simulink model "Final_System_Model_V2"  (R2018a)
settings: Solver=VariableStepAuto  StartTime=0  StopTime=inf  RelTol=1e-3
PreLoadFcn:
  | Ts_Power=1e-6;
  | Ts_Control=100e-6;
undefined symbols (not defined in the file): DiscIntNeverNeededParam, FC, FuelCellLoadFcn, gcbh, Ion, Lithium, sigbuilder_block, sps_rtmsupport
libraries: powerlib x20, simulink x10, fl_lib x8, nesl_utility x6, powerlib_meascontrol x5, electricdrivelib x1, spsFuelCellModel x1, re_lib x1
(part 1 of 4)
Description:
  | Copyright 2008-2017 The MathWorks, Inc.
settings Model: SimulationMode=accelerator  PacingRate=0.400000  Creator=MathWorks  LastModifiedBy=Mina
settings SolverCC: ZeroCrossControl=EnableAll  ZeroCrossAlgorithm=Adaptive  AlgebraicLoopSolver=LineSearch
settings DataIOCC: LimitDataPoints=on  SaveFormat=Array  SignalLoggingSaveFormat=ModelDataLogs  SignalLogging=off  DSMLogging=off
settings OptimizationCC: ExpressionDepthLimit=2147483647  LifeSpan=inf
settings DebuggingCC: SolverPrmCheckMsg=warning  FcnCallInpInsideContextMsg=warning  StateNameClashWarn=warning  SFUnexpectedBacktrackingDiag=warning  SFNoUnconditionalDefaultTransitionDiag=warning  SFExecutionAtInitializationDiag=none
settings HardwareCC: ProdBitPerPointer=32  ProdBitPerSizeT=32  ProdBitPerPtrDiffT=32  ProdLargestAtomicFloat=None  ProdIntDivRoundTo=Undefined  ProdEndianess=Unspecified  ProdWordSize=32  ProdHWDeviceType=32-bit Generic
settings ModelReferenceCC: PropagateSignalLabelsOutOfModel=off
settings CodeAppCC: StateflowObjectComments=on
settings GRTTargetCC: TargetLangStandard=C89/C90 (ANSI)  GeneratePreprocessorConditionals=Disable all  CombineOutputUpdateFcns=off  GRTInterface=on
settings ConfigComp: CovMetricSettings=dw  CovHtmlReporting=on  CovSaveCumulativeToWorkspaceVar=on  CovSaveSingleToWorkspaceVar=on  CovExternalEMLEnable=off  CovSFcnEnable=off
settings SimscapeCC: SimscapeNormalizeSystem=off

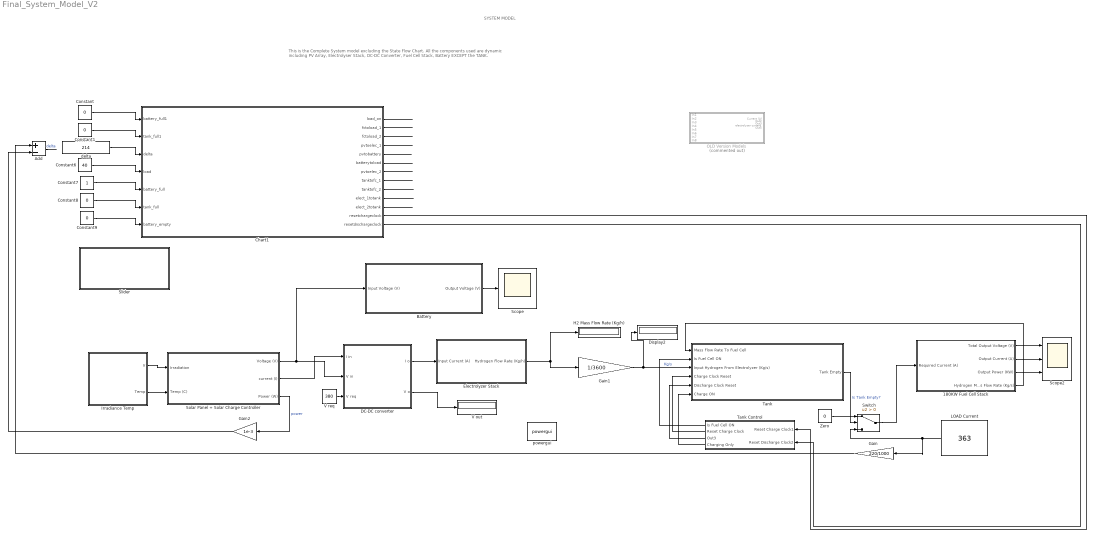
== system Final_System_Model_V2 ==
  note: SYSTEM MODEL
  note: This is the Complete System model excluding the State Flow Chart.
      |
      | All the components used are dynamic including PV Array, Electrolyser Stack, DC-DC Converter, Fuel Cell Stack, Battery EXCEPT the TANK.
  180KW Fuel Cell Stack : Subsystem
  Add : Sum  Inputs=+-
  Battery : Subsystem
  Chart1 : Stateflow chart  TreatAsAtomicUnit=on
  Constant{,1,8..9} (4 alike) : Constant  Value=0
  Constant6 : Constant  Value=40
  Constant7 : Constant
  DC-DC converter : Subsystem
  Display2 : Display
  Electrolyzer Stack : Subsystem
  Gain : Gain  Gain=220/1000
  Gain1 : Gain  Gain=1/3600
  Gain2 : Gain  Gain=1e-3
  H2 Mass Flow Rate (Kg/h) : Display
      settings: Format=short_e  Decimation=1000
  Irradiance Temp : Subsystem  Tag=STV Subsys  LoadFcn=sigbuilder_block('load');  StartFcn=sigbuilder_block('start');  StopFcn=sigbuilder_block('stop');  ClipboardFcn=sigbuilder_block('clipboard');  mask(Sigbuilder block){tuvar=[0:10]}
      mask help: Sigbuilder GUI
      mask init:
      | if ~strcmp(get_param(bdroot(gcbh),'SimulationStatus'),'stopped') tuvar = sigbuilder_block('maskInit'); end
      settings: CopyFcn=sigbuilder_block('copy');  DeleteFcn=sigbuilder_block('delete');  ModelCloseFcn=sigbuilder_block('modelClose');  PreSaveFcn=sigbuilder_block('preSave');  PauseFcn=sigbuilder_block('pause')  ContinueFcn=sigbuilder_block('continue')  NameChangeFcn=sigbuilder_block('namechange');  OpenFcn=sigbuilder_block('open',[216.75 189 451.5 323.25 ]);  CloseFcn=sigbuilder_block('close');
      mask Display: plot(0, 0, 100, 100,[2, 2, 32, 32, 2], [68, 8, 8, 68, 68],[32, 2], [38, 38], [32, 19, 2],[53, 60, 44], [32, 17, 17, 2],[16, 16, 31, 31]);txt = getActiveGroup(gcbh);text(2, 100, txt,'verticalAlignment', 'top');
  LOAD Current : Constant  Value=363
  OLD Version Models : Subsystem  Commented=on
  Scope : Scope
  Scope2 : Scope  NumInputPorts=3
  Slider : Subsystem  DialogController=hmiCreateDDGDialog  IsWebBlock=on  mask(MWDashboardBlock){webBlockId=9211a712-9074-4bf0-88da-f75de64371df, webBlockType=slider, ShowInLibBrowser=on, ShowInitialText=on, HMISrcModelName=Final_System_Model_V2}
      mask prompts: webBlockId "WebBlock Id"; webBlockType "WebBlock Type"; HMISrcModelName "Source Model"
      mask help: SimulinkHMI:dialogs:SliderDialogDesc
      mask Help: helpview([docroot '/mapfiles/simulink.map'], 'hmi_slider')
      mask Display:
      | if strcmp(get_param(bdroot(gcb),'BlockDiagramType'), 'library')
      |     image([(matlabroot) '/toolbox/simulink/hmi/icons/Slider.png']);
      | end
  Solar Panel + Solar Charge Controller : Subsystem
  Switch : Switch  Criteria=u2 > Threshold
  Tank : Subsystem
  Tank Control : Subsystem
  V out : Display
  V req : Constant  Value=380
  Zero : Constant  Value=0
  delta : Constant  Value=214
  powergui : powerlib/powergui  Priority=1  SimulationMode=Discrete  SampleTime=50e-6  frequency=60  Iterations=50  frequencyindice=0  Pbase=100e6  ErrMax=1e-4  UnitsV=kV  UnitsW=MW  buscounter=0  FunctionMessages=off  echomessages=off  EnableUseOfTLC=off  CurrentSourceSwitches=off  DisableSnubberDevices=off  DisableRonSwitches=off  DisableVfSwitches=off  DisplayEquations=off  SolverType=Tustin/Backward Euler (TBE)  Interpol=off  ExternalGateDelay=off  methode=off  Ts=100  x0status=blocks  SPID=off  SwTol=0  HookPort=off  RestoreLinks=warning  ResistiveCurrentMeasurement=off  Frange=[0:2:500]  Ylog=off  Xlog=on  ShowGrid=off  save=off  variable=ZData  structure=0  ZoomFFT=off  StartTime=0.0  cycles=1  DisplayStyle=1  fundamental=60  FreqAxis=off  MaxFrequency=1000  frequencyindicesteady=1  RmsSteady=1  display=off
  wires:
  Irradiance Temp/1(Ir) -> Solar Panel + Solar Charge Controller/1(Irradiation)
  Irradiance Temp/2(Temp) -> Solar Panel + Solar Charge Controller/2(Temp (C))
  Battery/1(Output Voltage (V)) -> Scope/1
  Electrolyzer Stack/1(Hydrogen Flow Rate (Kg/h)) -> H2 Mass Flow Rate (Kg/h)/1, Gain1/1
  180KW Fuel Cell Stack/1(Total Output Voltage (V)) -> Scope2/1
  180KW Fuel Cell Stack/2(Output Current (A)) -> Scope2/2
  180KW Fuel Cell Stack/3(Output Power (KW)) -> Scope2/3
  Gain1/1 -> Display2/1, Tank/3(Input Hydrogen From Electrolyzer (Kg/s))  "Kg/s"
  LOAD Current/1 -> Gain/1, Switch/3
  Solar Panel + Solar Charge Controller/3(Power (W)) -> Gain2/1  "power"
  180KW Fuel Cell Stack/4(Hydrogen Mass Flow Rate (Kg/s)) -> Tank/1(Mass Flow Rate To Fuel Cell)
  Tank/1(Tank Empty) -> Switch/2  "Is Tank Empty?"
  V req/1 -> DC-DC converter/3(V req)
  Solar Panel + Solar Charge Controller/1(Voltage (V)) -> DC-DC converter/2(V in), Battery/1(Input Voltage (V))
  DC-DC converter/1(I o) -> Electrolyzer Stack/1(Input Current (A))
  Solar Panel + Solar Charge Controller/2(current (I)) -> DC-DC converter/1(I in)
  DC-DC converter/2(V o) -> V out/1
  Tank Control/1(Is Fuel Cell ON) -> Tank/2(Is Fuel Cell ON)
  Tank Control/2(Reset Charge Clock) -> Tank/4(Charge Clock Reset)
  Tank Control/3(Out3) -> Tank/5(Discharge Clock Reset)
  Tank Control/4(Charging Only) -> Tank/6(Charge ON)
  Switch/1 -> 180KW Fuel Cell Stack/1(Required Current (A))
  Zero/1 -> Switch/1
  Gain/1 -> Add/1
  Gain2/1 -> Add/2
  Add/1 -> ?  "delta"
  Constant/1 -> Chart1/1(battery_full1)
  Constant1/1 -> Chart1/2(tank_full1)
  delta/1 -> Chart1/3(delta)
  Constant6/1 -> Chart1/4(load)
  Constant7/1 -> Chart1/5(battery_full)
  Constant8/1 -> Chart1/6(tank_full)
  Constant9/1 -> Chart1/7(battery_empty)
  Chart1/1(load_on) -> ?
  Chart1/2(fctoload_1) -> ?
  Chart1/3(fctoload_2) -> ?
  Chart1/4(pvtoelec_1) -> ?
  Chart1/5(pvtobattery) -> ?
  Chart1/6(batterytoload) -> ?
  Chart1/7(pvtoelec_2) -> ?
  Chart1/8(tanktofc_1) -> ?
  Chart1/9(tanktofc_2) -> ?
  Chart1/10(elect_1totank) -> ?
  Chart1/11(elect_2totank) -> ?
  Chart1/12(resetchargeclock) -> Tank Control/1(Reset Charge Clock1)
  Chart1/13(resetdischargeclock) -> Tank Control/2(Reset Discharge Clock2)

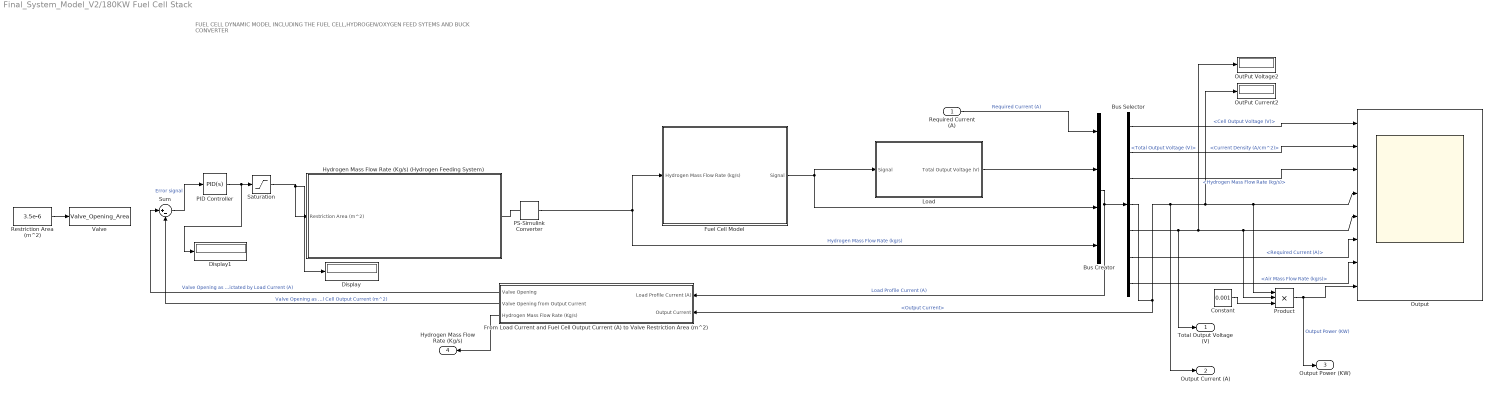
== system Final_System_Model_V2/180KW Fuel Cell Stack ==
  note: FUEL CELL DYNAMIC MODEL INCLUDING THE FUEL CELL,HYDROGEN/OXYGEN FEED SYTEMS AND BUCK CONVERTER
  Required Current (A) : Inport
  Bus Creator : BusCreator  Inputs=4
  Bus Selector : BusSelector  OutputSignals=|
      | signal3.Cell Output Voltage (V),signal3.Current Density (A/cm^2),Hydrogen Mass Flow Rate (kg/s),signal3.Output Current,Total Output Voltage (V),Required Current
      | (A),signal3.Air Mass Flow Rate (kg/s)
  Constant : Constant  Value=0.001
  Display : Display
  Display1 : Display
  From Load Current and Fuel Cell Output Current (A) to Valve Restriction Area (m^2) : Subsystem
  Fuel Cell Model : Subsystem  mask(Fuel Cell Model){Temperature_c=80, Hydrogen_Pressure_atm=8, Air_Pressure_atm=8, Number_of_cells=208, Cell_Area_cm_squared=4397.14, Alpha_charge_Transfer_Coefficient=0.5, Exchange_Current_Density_i0=0.00000012246, Internal_Resistance_r=0.019, Amplification_Constant_Alpha1=0.085, Limiting_Current_Density_i_l=2, Mass_Transport_Limit_k=1.1, Dynamic_Response=[5 1]}
      mask prompts: Temperature_c "Temperature (c)"; Hydrogen_Pressure_atm "Hydrogen Pressure (atm)"; Air_Pressure_atm "Air Pressure (atm)"; Number_of_cells "Number Of Cells"; Cell_Area_cm_squared "Cell Area (cm^2)"; Alpha_charge_Transfer_Coefficient "Alpha (Charge Transfer Coefficient)"; Exchange_Current_Density_i0 "Exchange Current Density (i_0)(A/cm^2)"; Internal_Resistance_r "Internal Resistance (r)(Ohm)"; Amplification_Constant_Alpha1 "Amplification Constant (Alpha1)"; Limiting_Current_Density_i_l "Limiting Current Density (i_L)(A/cm^2)"; Mass_Transport_Limit_k "Mass Transport Limit (k)"; Dynamic_Response "Cell Dynamic Response (s)"
      mask help:
      | This is a mathematical Fuel Cell dynamic model. It operates under the Following Assumptions:
      | 1-The model is dynamic ,ie, it models the fuel cell behavior with respect to time.
      | 2-Fuel Cell Temperature is Constant.
      | 3-No Excess Hydrogen ,ie, Every Hydrogen molecule that enters the fuel cell Stack reacts to produce electricity.
      | 4-No excess Air.
      | 5-Concentration Losses are not calculated in the Model as we will never approach this region during operation.
      mask TypeOptions Temperature_c:
      | Stack Temperature
      | (C)/Value
      mask TypeOptions Hydrogen_Pressure_atm: Hydrogen Pressure (atm)/Value
      mask TypeOptions Air_Pressure_atm: Air Pressue (atm)/Value
      mask TypeOptions Number_of_cells: Number of Cells/Value
      mask TypeOptions Cell_Area_cm_squared:
      | Cell Area
      | (cm^2)/Value
      mask TypeOptions Alpha_charge_Transfer_Coefficient:
      | From Current Density (A//cm^2)
      | To
      | Overvoltages (V)/Activation Overvoltage/Alpha
      | Charge Transfer Coefficient1/Value
      mask TypeOptions Exchange_Current_Density_i0:
      | From Current Density (A//cm^2)
      | To
      | Overvoltages (V)/Activation Overvoltage/Reference Exchange Current Density
      | (I_0)1/Value
      mask TypeOptions Internal_Resistance_r:
      | From Current Density (A//cm^2)
      | To
      | Overvoltages (V)/Ohmic Overvoltage/Internal Resistance
      | (r)/Value
      mask TypeOptions Amplification_Constant_Alpha1:
      | From Current Density (A//cm^2)
      | To
      | Overvoltages (V)/Concentration Overvoltage/Amplification Constant
      | Alpha2/Value
      mask TypeOptions Limiting_Current_Density_i_l:
      | From Current Density (A//cm^2)
      | To
      | Overvoltages (V)/Concentration Overvoltage/Limiting Current
      | (i_L)1/Value
      mask TypeOptions Mass_Transport_Limit_k:
      | From Current Density (A//cm^2)
      | To
      | Overvoltages (V)/Concentration Overvoltage/Mass Transport Constant
      | (K)1/Value
      mask TypeOptions Dynamic_Response: Cell dynamic/Denominator
      mask DialogControl Operating_Conditions Prompt: Operating Conditions
      mask DialogControl Fuel_Cell_Parameters Prompt: Fuel Cell Parameters
      mask Display: image(imread('power_fuelcell.png'));port_label('output',1,'m');
  Hydrogen Mass Flow Rate (Kg/s) (Hydrogen Feeding System) : Subsystem
  Load : Subsystem
  OutPut Current2 : Display
  OutPut Voltage2 : Display
  "Output " : Scope  NumInputPorts=8
  PID Controller : simulink/Continuous/PID Controller  Controller=PID  TimeDomain=Continuous-time  SampleTime=-1  IntegratorMethod=Forward Euler  FilterMethod=Forward Euler  Form=Parallel  UseFilter=on  ControllerParametersSource=internal  P=0.5  I=0.7  D=0.01  N=100  InitialConditionSource=internal  InitialConditionForIntegrator=0  InitialConditionForFilter=0  ExternalReset=none  LimitOutput=on  UpperSaturationLimit=2.7e-5  LowerSaturationLimit=-inf  LinearizeAsGain=on  AntiWindupMode=none  Kb=1  TrackingMode=off  Kt=1  PParamMin=[]  PParamMax=[]  IParamMin=[]  IParamMax=[]  DParamMin=[]  DParamMax=[]  NParamMin=[]  NParamMax=[]  KbParamMin=[]  KbParamMax=[]  KtParamMin=[]  KtParamMax=[]  POutMin=[]  POutMax=[]  IOutMin=[]  IOutMax=[]  DOutMin=[]  DOutMax=[]  NOutMin=[]  NOutMax=[]  KbOutMin=[]  KbOutMax=[]  KtOutMin=[]  KtOutMax=[]  IntegratorOutMin=[]  IntegratorOutMax=[]  FilterOutMin=[]  FilterOutMax=[]  SumOutMin=[]  SumOutMax=[]  SumI1OutMin=[]  SumI1OutMax=[]  SumI2OutMin=[]  SumI2OutMax=[]  SumI3OutMin=[]  SumI3OutMax=[]  SumDOutMin=[]  SumDOutMax=[]  SaturationOutMin=[]  SaturationOutMax=[]  IntegratorContinuousStateAttributes=''  IntegratorStateMustResolveToSignalObject=off  IntegratorRTWStateStorageClass=Auto  FilterContinuousStateAttributes=''  FilterStateMustResolveToSignalObject=off  FilterRTWStateStorageClass=Auto  DifferentiatorICPrevScaledInput=0  DifferentiatorOutMin=[]  DifferentiatorOutMax=[]  FilterDiffOutCoefMin=[]  FilterDiffOutCoefMax=[]  SumDenOutMin=[]  SumDenOutMax=[]  SumNumOutMin=[]  SumNumOutMax=[]  ReciprocalOutMin=[]  ReciprocalOutMax=[]  DivideOutMin=[]  DivideOutMax=[]  TunerSelectOption=Transfer Function Based (PID Tuner App)
  PS-Simulink Converter : nesl_utility/PS-Simulink Converter  PhysicalDomain=network_engine_domain  SubClassName=ps_output  LeftPortType=input  RightPortType=output  PseudoPeriodic=off  Frequencies=[]  Unit=1  AffineConversion=off
  Product : Product  Inputs=3
  "Restriction Area (m^2) " : Constant  Value=3.5e-6  VectorParams1D=off
  Saturation : Saturate  UpperLimit=2.7e-5  LowerLimit=0
  Sum : Sum  Inputs=|+-
  Valve : ToWorkspace  VariableName=Valve_Opening_Area  SaveFormat=Timeseries  SampleTime=-1
  Total Output Voltage (V) : Outport
  Output Current (A) : Outport  Port=2
  Output Power (KW) : Outport  Port=3
  Hydrogen Mass Flow Rate (Kg/s) : Outport  Port=4
  wires:
  Bus Selector/7 -> "Output "/7  "<Air Mass Flow Rate (kg/s)>"
  Required Current (A)/1 -> Bus Creator/1  "Required Current (A)"
  Product/1 -> Output Power (KW)/1, "Output "/8  "Output Power (KW)"
  From Load Current and Fuel Cell Output Current (A) to Valve Restriction Area (m^2)/2(Valve Opening from Output Current) -> Sum/2  "Valve Opening as dictated by Fuel Cell Output Current (m^2)"
  Bus Selector/4 -> Output Current (A)/1, OutPut Current2/1, Product/1, "Output "/4, From Load Current and Fuel Cell Output Current (A) to Valve Restriction Area (m^2)/2(Output Current)  "<Output Current>"
  PS-Simulink Converter/1 -> Fuel Cell Model/1(Hydrogen Mass Flow Rate (kg/s)), Bus Creator/4  "Hydrogen Mass Flow Rate (kg/s)"
  Bus Selector/1 -> "Output "/1  "<Cell Output Voltage (V)>"
  Constant/1 -> Product/3
  Bus Creator/1 -> From Load Current and Fuel Cell Output Current (A) to Valve Restriction Area (m^2)/1(Load Profile Current (A)), Bus Selector/1  "Load Profile Current (A)"
  Bus Selector/2 -> "Output "/2  "<Current Density (A/cm^2)>"
  Bus Selector/5 -> Total Output Voltage (V)/1, OutPut Voltage2/1, Product/2, "Output "/5  "<Total Output Voltage (V)>"
  Fuel Cell Model/1(Signal) -> Bus Creator/3, Load/1(Signal)
  Load/1(Total Output Voltage (V)) -> Bus Creator/2
  Bus Selector/3 -> "Output "/3  "<Hydrogen Mass Flow Rate (kg/s)>"
  Sum/1 -> PID Controller/1  "Error signal"
  From Load Current and Fuel Cell Output Current (A) to Valve Restriction Area (m^2)/1(Valve Opening) -> Sum/1  "Valve Opening as dictated by Load Current (A)"
  Saturation/1 -> Display/1, Hydrogen Mass Flow Rate (Kg/s) (Hydrogen Feeding System)/1(Restriction Area (m^2))
  "Restriction Area (m^2) "/1 -> Valve/1
  Bus Selector/6 -> "Output "/6  "<Required Current (A)>"
  PID Controller/1 -> Saturation/1, Display1/1
  From Load Current and Fuel Cell Output Current (A) to Valve Restriction Area (m^2)/3(Hydrogen Mass Flow Rate (Kg/s)) -> Hydrogen Mass Flow Rate (Kg/s)/1
  connections:
  PS-Simulink Converter/LConn1 -- Hydrogen Mass Flow Rate (Kg/s) (Hydrogen Feeding System)/RConn1

== system Final_System_Model_V2/Battery ==
  Input Voltage (V) : Inport
  Battery : electricdrivelib/Extra Sources/Battery  BatType=Lithium-Ion  ShowTempParam=off  ThermalPreset=no  ShowAgeParam=off  NomV=48  NomQ=2000  SOC=100  Batt_Tr=30  PresetModel=on  MaxQ=2000  MinV=36  FullV=55.8714  Dis_rate=869.5652  R=0.00024  Normal_OP=1808.6957  expZone="[51.8585      98.2609]"  current=[6.5 13 32.5]  Units=Time  Tci=20  NomT=20  T2=-30  MaxQ2=4.8  FullV2=7.1  Normal_OP2=5.655  expZone2="[6.58           1]"  Rca=0.6  ti=2000  Dp=0  Neq0=0  Tsim=1e6  Ta1=25  Qeol=5.4*0.9  Reol=0.013333*1.2  Char_age=[2.3478, 3]  Dis_age=[2.3478, 10]  N1=1500  N2=10500  N3=1000  N4=1400  Ta2=45  N5=950
  Bus Selector : BusSelector  OutputSignals=SOC (%),Current (A),Voltage (V)
  Constant : Constant  Value=100
  Controlled Voltage Source1 : powerlib/Electrical Sources/Controlled Voltage Source  Initialize=on  Source_Type=AC  Amplitude=0  Phase=0  Frequency=0  Measurements=None
  Scope : Scope  NumInputPorts=3
  Scope1 : Scope
  Voltage Measurement : powerlib/Measurements/Voltage Measurement  PhasorSimulation=off  OutputType=Complex  PSBequivalent=0
  Output Voltage (V) : Outport
  wires:
  Bus Selector/1 -> Scope/1  "<SOC (%)>"
  Bus Selector/2 -> Scope/2  "<Current (A)>"
  Bus Selector/3 -> Scope/3  "<Voltage (V)>"
  Input Voltage (V)/1 -> ?
  Battery/1 -> Bus Selector/1
  Voltage Measurement/1 -> Scope1/1
  Constant/1 -> Controlled Voltage Source1/1
  connections:
  Battery/LConn1 -- Voltage Measurement/LConn1 -- Controlled Voltage Source1/RConn1
  Voltage Measurement/LConn2 -- Controlled Voltage Source1/LConn1 -- Battery/LConn2

== system Final_System_Model_V2/DC-DC converter ==
  I in : Inport
  V in : Inport  Port=2
  V req : Inport  Port=3
  Subsystem : Subsystem
  duty cycle : Subsystem
  I o : Outport
  V o : Outport  Port=2
  wires:
  V req/1 -> duty cycle/2(V req)
  Subsystem/2(V o) -> V o/1
  V in/1 -> duty cycle/1(V in), Subsystem/3(V in)
  [duty_cycle] -> Subsystem/1(duty cycle)
  Subsystem/1(I o) -> I o/1
  I in/1 -> Subsystem/2(I in)

== system Final_System_Model_V2/Electrolyzer Stack ==
  Input Current (A) : Inport
  Divide : Product  Inputs=*/
  Gain : Gain  Gain=3.6
  H2 flow rate in kg/h : Scope
  Saturation : Saturate  UpperLimit=1.2  LowerLimit=0
  T : Constant  Value=333
  area in cm^2 : Constant  Value=428
  electrolyser stack : Subsystem
  voltage : Scope
  Hydrogen Flow Rate (Kg/h) : Outport
  wires:
  Saturation/1 -> electrolyser stack/2(In2)  "Current Density (A/cm^2)"
  electrolyser stack/2(Out3) -> Gain/1  "H2 flow rate in g/s"
  T/1 -> electrolyser stack/1(In1)
  electrolyser stack/1(Out1) -> voltage/1
  Input Current (A)/1 -> Divide/1
  area in cm^2/1 -> Divide/2
  Divide/1 -> Saturation/1
  Gain/1 -> Hydrogen Flow Rate (Kg/h)/1, H2 flow rate in kg/h/1  "H2 flow rate in kg/h"

== system Final_System_Model_V2/Irradiance Temp ==
  Demux : Demux  Tag=STV Demux  Outputs=2
  FromWs : FromWorkspace  Tag=STV FromWs  VariableName=tuvar  SampleTime=0
      SigBuilderData=|
      | common.afterFinalStr = 'Extrapolate'
      | common.sampleTime = '0'
      | dataSet(1).timeRange = [0 2]
      | dataSet(1).name = 'Constant Irradiance'
      | dataSet(2).timeRange = [0 2]
      | dataSet(2).name = 'Step Irradiance'
      | dataSet(3).timeRange = [0 3]
      | dataSet(3).name = 'Ramp-up/down Irradiance'
      | sbobj.Groups(1).Name = 'Constant Irradiance'
      | sbobj.Groups(1).Signals(1).Name = 'Ir'
      | sbobj.Groups(1).Signals(1).XData = [0 2]
      | sbobj.Groups(1).Signals(1).YData = [1000 1000]
      | sbobj.Groups(1).Signals(2).Name = 'Temp'
      | sbobj.Groups(1).Signals(2).XData = [0 1 1 2]
      | sbobj.Groups(1).Signals(2).YData = [0 0 1 1]
      | sbobj.Groups(1).TimeRange = [0 2]
      | sbobj.Groups(2).Name = 'Step Irradiance'
      | sbobj.Groups(2).Signals(1).Name = 'Ir'
      | sbobj.Groups(2).Signals(1).XData = [0 0.252 0.252 2]
      | sbobj.Groups(2).Signals(1).YData = [600 600 1000 1000]
      | sbobj.Groups(2).Signals(2).Name = 'Temp'
      | sbobj.Groups(2).Signals(2).XData = [0 1 1 2]
      | sbobj.Groups(2).Signals(2).YData = [0 0 1 1]
      | sbobj.Groups(2).TimeRange = [0 2]
      | sbobj.Groups(3).Name = 'Ramp-up/down Irradiance'
      | sbobj.Groups(3).Signals(1).Name = 'Ir'
      | sbobj.Groups(3).Signals(1).XData = [0 0.6 1.1 1.2 1.7 3]
      | sbobj.Groups(3).Signals(1).YData = [1000 1000 1000 1000 1000 1000]
      | sbobj.Groups(3).Signals(2).Name = 'Temp'
      | sbobj.Groups(3).Signals(2).XData = [0 2 2.1 3]
      | sbobj.Groups(3).Signals(2).YData = [25 25 25 25]
      | sbobj.Groups(3).TimeRange = [0 3]
  Ir : Outport  Tag=STV Outport
  Temp : Outport  Tag=STV Outport  Port=2
  wires:
  Demux/1 -> Ir/1
  FromWs/1 -> Demux/1
  Demux/2 -> Temp/1

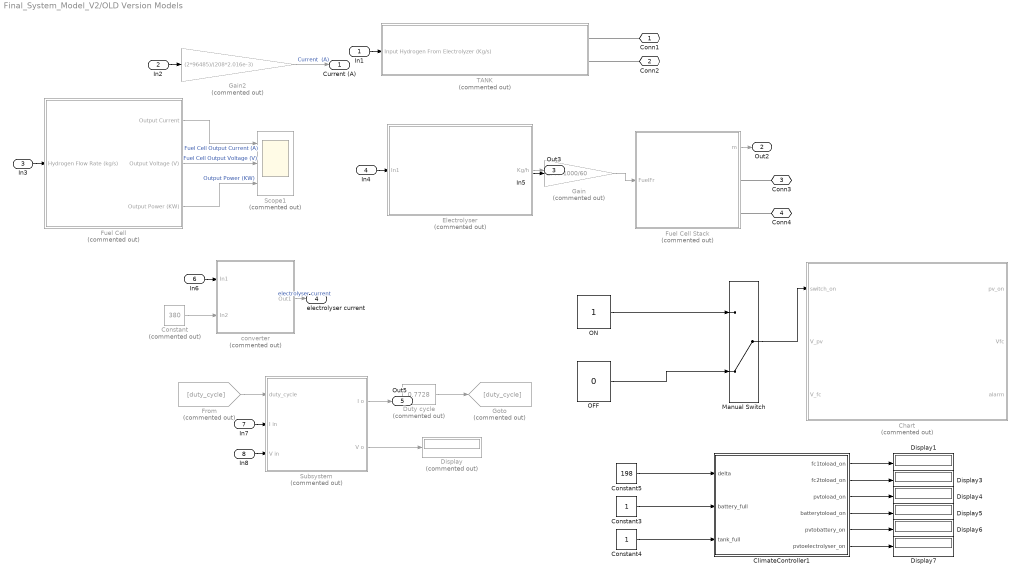
== system Final_System_Model_V2/OLD Version Models ==
  In1 : Inport
  In2 : Inport  Port=2
  In3 : Inport  Port=3
  In4 : Inport  Port=4
  In5 : Inport  Port=5
  In6 : Inport  Port=6
  In7 : Inport  Port=7
  In8 : Inport  Port=8
  Chart : Stateflow chart  Commented=on  TreatAsAtomicUnit=on
  ClimateController1 : Truth Table  TreatAsAtomicUnit=on
  Constant : Constant  Commented=on  Value=380
  Constant3 : Constant
  Constant4 : Constant
  Constant5 : Constant  Value=198
  Display : Display  Commented=on
  Display{1,3..7} (6 alike) : Display
  Duty cycle : Constant  Commented=on  Value=0.7728
  Electrolyser : Subsystem  Commented=on
  From : From  Commented=on  GotoTag=duty_cycle
  Fuel Cell : Subsystem  Commented=on
  Fuel Cell Stack : Subsystem  Commented=on  AncestorBlock=electricdrivelib/Extra Sources/Fuel Cell Stack  DialogController=POWERSYS.PowerSysDialog  LoadFcn=sps_rtmsupport('LoadFcn',gcbh);FuelCellLoadFcn(gcb)  StartFcn=sps_rtmsupport('StartFcn',gcbh);  StopFcn=sps_rtmsupport('StopFcn',gcbh);  mask(Fuel Cell Stack){PresetModel=PEMFC - 6 kW - 45 Vdc, FcType=0, Detailed=Detailed, Eoc=[65,63], NomVI=[133.3,45], EndVI=[225,37], Nc=65, n=55, TOp=65, AirFr=300, SuppPress=[1.5,1], Comp=[99.95,21,1], SignX=off, SignY=off, FlowRateH2=on, FlowRateAir=off, SystemTemp=off, SystemPH2=off, SystemPAir=off, FCDyn=off, FC_tau=1, Peak_O2=80, V_Under=10}
      mask prompts: PresetModel "Preset model:"; FcType "Fuel Cell type:"; Detailed "Model detail Level:"; Eoc "Voltage at 0A and 1A [V_0(V), V_1(V)]"; NomVI "Nominal operating point [Inom(A), Vnom(V)]"; EndVI "Maximum operating point [Iend(A), Vend(V)]"; Nc "Number of cells"; n "Nominal stack efficiency (%)"; TOp "Operating temperature (Celsius)"; AirFr "Nominal Air flow rate (lpm)"; SuppPress "Nominal supply pressure [Fuel (bar), Air (bar)]"; Comp "Nominal composition (%) [H2 O2 H2O(Air)]"; SignX "Fuel  composition [x_H2(%)]"; SignY "Oxidant composition [y_O2(%)]"; FlowRateH2 "Fuel flow rate [FuelFr(lpm)]"; FlowRateAir "Air flow rate [AirFr(lpm)]"; SystemTemp "System Temperature [T(Kelvin)]"; SystemPH2 "Fuel supply pressure [Pfuel(bar)]"; SystemPAir "Air supply pressure [PAir(bar)]"; FCDyn "Specify Fuel Cell Dynamics?"; FC_tau "Fuel Cell response time (sec)"; Peak_O2 "Peak O2 utilization (%)"; V_Under "Voltage undershoot (V) @ peak O2 utilization"
      mask help:
      | Implements a generic hydrogen fuel cell model which allows the simulation for the following types of cells:
      | - Proton Exchange Membrane Fuel Cell (PEMFC)
      | - Solid Oxide Fuel Cell (SOFC)
      | - Alkaline Fuel Cell (AFC)
      mask init:
      | block = gcb;
      | %% DO NOT CHANGE THIS ORDER
      | FuelCellCback(block,'Inputs')
      | [FC, WantBlockChoice, Ts] = FuelCellInit(block,Eoc,NomVI,EndVI,Nc,n,TOp,AirFr,SuppPress,Comp,FlowRateH2,FlowRateAir);
      | powericon('SetInternalModels','set',block,WantBlockChoice);
      settings: CopyFcn=sps_rtmsupport('CopyFcn',gcbh);  DeleteFcn=sps_rtmsupport('DeleteFcn',gcbh);  UndoDeleteFcn=sps_rtmsupport('UndoDeleteFcn',gcbh);  ModelCloseFcn=sps_rtmsupport('ModelCloseFcn',gcbh);  PreSaveFcn=sps_rtmsupport('PreSaveFcn',gcbh);  PostSaveFcn=sps_rtmsupport('PostSaveFcn',gcbh);  NameChangeFcn=sps_rtmsupport('NameChangeFcn',gcbh);  PreCopyFcn=sps_rtmsupport('PreCopyFcn',gcbh);  OpenFcn=sps_rtmsupport('OpenFcn',gcbh, [1 2 3 13 14 15 16 17 18 19 20]);  CloseFcn=sps_rtmsupport('CloseFcn',gcbh);  PreDeleteFcn=sps_rtmsupport('PreDeleteFcn',gcbh);
      mask Help: helpview(psbhelp)
      mask TypeOptions PresetModel: No (User-Defined) | PEMFC - 1.26 kW - 24 Vdc | PEMFC - 6 kW - 45 Vdc | PEMFC - 50 kW - 625 Vdc | AFC - 2.4 kW - 48 Vdc | SOFC - 3 kW - 100 Vdc | SOFC - 25 kW - 630 Vdc
      mask Callback PresetModel: FuelCellCback(gcb,'Preset')
      mask TypeOptions Detailed: Simplified | Detailed
      mask Callback Detailed: FuelCellCback(gcb,'Visibilities')
      mask Callback FlowRateAir: FuelCellCback(gcb,'Visibilities')
      mask Callback FCDyn: FuelCellCback(gcb,'Visibilities')
      mask DialogControl ParameterTabVar0 Prompt: Parameters
      mask DialogControl plot_graph Prompt: Plot V_I characteristic
      mask DialogControl plot_graph Callback: FuelCellCback(gcb,'PlotGraph');
      mask DialogControl ViewParam Prompt: View Cell parameters
      mask DialogControl ViewParam Callback: FuelCellCback(gcb,'ViewParam');
      mask DialogControl ParameterTabVar01 Prompt: Signal variation
      mask DialogControl ParameterTabVar012 Prompt: Fuel Cell Dynamics
      mask Display: image(imread('power_fuelcell.png'));
  Gain : Gain  Commented=on  Gain=2.44*1000/60
  Gain2 : Gain  Commented=on  Gain=(2*96485)/(208*2.016e-3)
  Goto : Goto  Commented=on  GotoTag=duty_cycle
  Manual Switch : ManualSwitch  CurrentSetting=0
  OFF : Constant  Value=0
  ON : Constant
  Scope1 : Scope  Commented=on  NumInputPorts=3
  Subsystem : Subsystem  Commented=on
  TANK : Subsystem  Commented=on
  converter : Subsystem  Commented=on
  Conn1 : PMIOPort  Side=Right
  Conn2 : PMIOPort  Port=2  Side=Right
  Conn3 : PMIOPort  Port=3  Side=Right
  Conn4 : PMIOPort  Port=4  Side=Right
  Current (A) : Outport
  Out2 : Outport  Port=2
  Out3 : Outport  Port=3
  electrolyser current : Outport  Port=4
  Out5 : Outport  Port=5
  wires:
  Fuel Cell/1(Output Current) -> Scope1/1  "Fuel Cell Output Current (A)"
  From/1 -> Subsystem/1(duty_cycle)
  Fuel Cell/2(Output Voltage (V)) -> Scope1/2  "Fuel Cell Output Voltage (V)"
  Fuel Cell/3(Output Power (KW)) -> Scope1/3  "Output Power (KW)"
  Subsystem/1(I o) -> Out5/1
  Duty cycle/1 -> Goto/1
  Constant/1 -> converter/2(In2)
  Subsystem/2(V o) -> Display/1
  In5/1 -> Gain/1
  Gain/1 -> Fuel Cell Stack/1(FuelFr)
  In7/1 -> Subsystem/2(I in)
  Gain2/1 -> Current (A)/1  "Current  (A)"
  In2/1 -> Gain2/1
  In1/1 -> TANK/1(Input Hydrogen From Electrolyzer (Kg/s))
  Electrolyser/1(Kg/h) -> Out3/1
  converter/1(Out1) -> electrolyser current/1  "electrolyser current"
  In6/1 -> converter/1(In1)
  In4/1 -> Electrolyser/1(In1)
  In8/1 -> Subsystem/3(V in)
  Fuel Cell Stack/1(m) -> Out2/1
  In3/1 -> Fuel Cell/1("Hydrogen Flow Rate (kg/s) ")
  Constant5/1 -> ClimateController1/1(delta)
  ClimateController1/2(fc2toload_on) -> Display3/1
  ClimateController1/5(pvtobattery_on) -> Display6/1
  ClimateController1/6(pvtoelectrolyser_on) -> Display7/1
  Constant3/1 -> ClimateController1/2(battery_full)
  Constant4/1 -> ClimateController1/3(tank_full)
  ON/1 -> Manual Switch/1
  ClimateController1/1(fc1toload_on) -> Display1/1
  ClimateController1/4(batterytoload_on) -> Display5/1
  OFF/1 -> Manual Switch/2
  ClimateController1/3(pvtoload_on) -> Display4/1
  Manual Switch/1 -> Chart/1(switch_on)
  connections:
  Fuel Cell Stack/RConn1 -- Conn3/RConn1
  Fuel Cell Stack/RConn2 -- Conn4/RConn1
  TANK/RConn1 -- Conn1/RConn1
  TANK/RConn2 -- Conn2/RConn1

== system Final_System_Model_V2/Slider ==

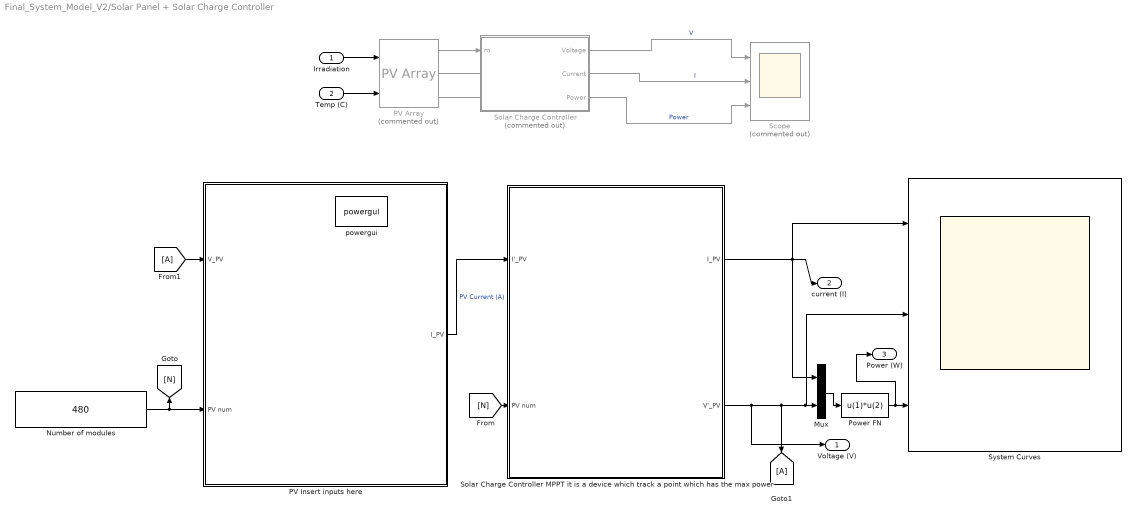
== system Final_System_Model_V2/Solar Panel + Solar Charge Controller ==
  Irradiation : Inport
  Temp (C) : Inport  Port=2
  Mux : Mux  Inputs=2
  Number of modules : Constant  Value=480
  PV Insert inputs here : Subsystem
      mask Display: image('C:\Users\Kimo Store\Desktop\PV Simulink\pva.jpg');
  PV Array : re_lib/Solar/PV Array  Commented=on  Npar=240  Nser=2  PlotType=array @ 1000 W/m2 & specified temperatures  S_vec="[ 1000  250 ]"  Temp_C_vec="[0 25 50  ]"  ModuleName=SunPower SPR-X21-345-COM  PlotWhenSelected=off  Pm=344.946  Ncell=96  Voc=68.2  Isc=6.39  Vm=57.3  Im=6.02  beta_Voc_pc=-0.356  alpha_Isc_pc=0.07  beta_Voc=-0.24279  alpha_Isc=0.004473  IL=6.3928  I0=1.9084e-10  nI=1.1415  Rsh=884.5543  Rs=0.39387  BAL=on  Tc=5e-7  Tfilter=5e-5
  "Power FN " : Fcn  Expr=u(1)*u(2)
  Scope : Scope  Commented=on  NumInputPorts=3
  Solar Charge Controller : Subsystem  Commented=on
  Solar Charge Controller MPPT it is a device which track a point which has the max power : Subsystem
  System Curves : Scope  NumInputPorts=3
  powergui : powerlib/powergui  Priority=1  SimulationMode=Continuous  SampleTime=50e-6  frequency=60  Iterations=50  frequencyindice=0  Pbase=100e6  ErrMax=1e-4  UnitsV=kV  UnitsW=MW  buscounter=0  FunctionMessages=off  echomessages=off  EnableUseOfTLC=off  CurrentSourceSwitches=off  DisableSnubberDevices=off  DisableRonSwitches=off  DisableVfSwitches=off  DisplayEquations=off  SolverType=Tustin/Backward Euler (TBE)  Interpol=off  ExternalGateDelay=off  methode=off  Ts=100  x0status=blocks  SPID=on  SwTol=0  HookPort=off  RestoreLinks=warning  ResistiveCurrentMeasurement=off  Frange=[0:2:500]  Ylog=off  Xlog=on  ShowGrid=off  save=off  variable=ZData  structure=0  ZoomFFT=off  StartTime=0.0  cycles=1  DisplayStyle=1  fundamental=60  FreqAxis=off  MaxFrequency=1000  frequencyindicesteady=1  RmsSteady=1  display=off
  Voltage (V) : Outport
  current (I) : Outport  Port=2
  Power (W) : Outport  Port=3
  wires:
  PV Array/1 -> Solar Charge Controller/1(m)
  Solar Charge Controller/3(Power) -> Scope/3  "Power"
  Irradiation/1 -> PV Array/1
  Temp (C)/1 -> PV Array/2
  Solar Charge Controller/2(Current) -> Scope/2  "I"
  Solar Charge Controller/1(Voltage) -> Scope/1  "V"
  PV Insert inputs here/1(I_PV) -> Solar Charge Controller MPPT it is a device which track a point which has the max power/1(I'_PV)  "PV Current (A)"
  [N] -> Solar Charge Controller MPPT it is a device which track a point which has the max power/2(PV num)
  Solar Charge Controller MPPT it is a device which track a point which has the max power/1(I_PV) -> current (I)/1, Mux/1, System Curves/1
  [A] -> PV Insert inputs here/1(V_PV)
  "Power FN "/1 -> Power (W)/1, System Curves/3
  Number of modules/1 -> PV Insert inputs here/2(PV num), [N]
  Mux/1 -> "Power FN "/1
  Solar Charge Controller MPPT it is a device which track a point which has the max power/2("V'_PV ") -> Voltage (V)/1, [A], System Curves/2, Mux/2
  connections:
  PV Array/RConn1 -- Solar Charge Controller/LConn1
  PV Array/RConn2 -- Solar Charge Controller/LConn2

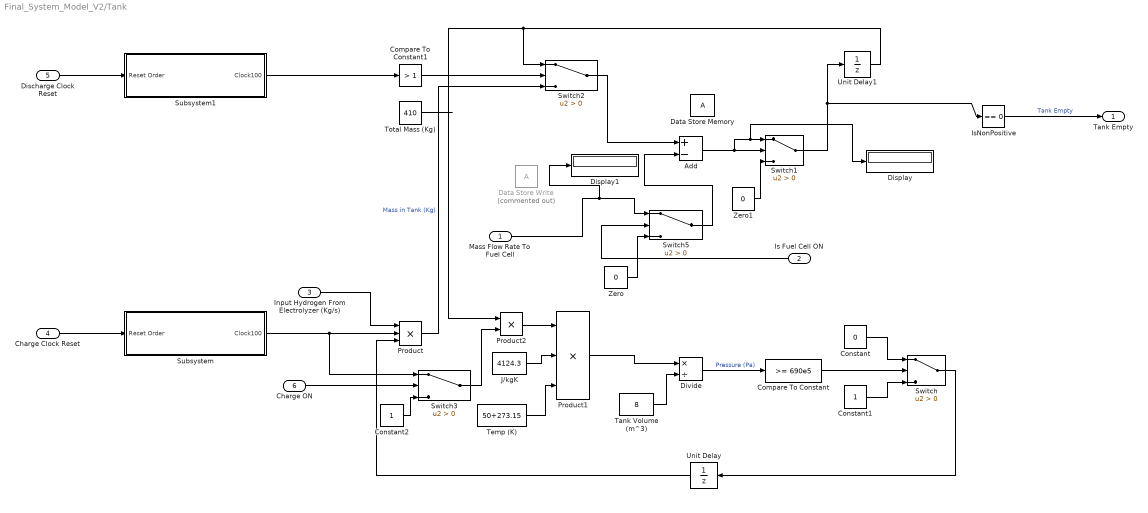
== system Final_System_Model_V2/Tank ==
  Mass Flow Rate To Fuel Cell : Inport
  Is Fuel Cell ON : Inport  Port=2
  Input Hydrogen From Electrolyzer (Kg/s) : Inport  Port=3
  Charge Clock Reset : Inport  Port=4
  Discharge Clock Reset : Inport  Port=5
  Charge ON : Inport  Port=6
  Add : Sum  Inputs=+-
  Compare To Constant : simulink/Logic and Bit Operations/Compare To Constant  relop=>=  const=690e5  OutDataTypeStr=boolean
  Compare To Constant1 : simulink/Logic and Bit Operations/Compare To Constant  relop=>  const=1  OutDataTypeStr=boolean
  Constant : Constant  Value=0
  Constant1 : Constant
  Constant2 : Constant
  Data Store Memory : DataStoreMemory  ReadBeforeWriteMsg=warning  WriteAfterWriteMsg=warning  WriteAfterReadMsg=warning  ShowAdditionalParam=off
  Data Store Write : DataStoreWrite  Commented=on  DataStoreElements=A
  Display : Display
  Display1 : Display
  Divide : Product  Inputs=*/
  IsNonPositive : simulink/Logic and Bit Operations/Compare To Zero  relop===  OutDataTypeStr=boolean
  J/kgK : Constant  Value=4124.3
  Product : Product  Inputs=3
  Product1 : Product  Inputs=3
  Product2 : Product
  Subsystem : Subsystem
  Subsystem1 : Subsystem
  Switch{,1..3,5} (5 alike) : Switch  Criteria=u2 > Threshold
  Tank Volume (m^3) : Constant  Value=8
  Temp (K) : Constant  Value=50+273.15
  Total Mass (Kg) : Constant  Value=410
  Unit Delay : UnitDelay  SampleTime=-1
  Unit Delay1 : UnitDelay  SampleTime=-1
  Zero : Constant  Value=0
  Zero1 : Constant  Value=0
  Tank Empty : Outport
  wires:
  Switch/1 -> Unit Delay/1
  Product1/1 -> Divide/1
  Add/1 -> Display/1, Switch1/1, Switch1/2
  Switch5/1 -> Add/2
  Divide/1 -> Compare To Constant/1  "Pressure (Pa)"
  Tank Volume (m^3)/1 -> Divide/2
  Temp (K)/1 -> Product1/3
  Switch1/1 -> IsNonPositive/1, Unit Delay1/1
  Charge Clock Reset/1 -> Subsystem/1(Reset Order)
  J/kgK/1 -> Product1/2
  Switch2/1 -> Add/1
  Constant1/1 -> Switch/3
  Compare To Constant1/1 -> Switch2/2
  Subsystem1/1(Clock100) -> Compare To Constant1/1
  Subsystem/1(Clock100) -> Switch3/1, Product/2
  Is Fuel Cell ON/1 -> Switch5/2
  IsNonPositive/1 -> Tank Empty/1  "Tank Empty"
  Compare To Constant/1 -> Switch/2
  Constant/1 -> Switch/1
  Zero/1 -> Switch5/3
  Input Hydrogen From Electrolyzer (Kg/s)/1 -> Product/1
  Mass Flow Rate To Fuel Cell/1 -> Display1/1, Switch5/1
  Unit Delay/1 -> Product/3
  Zero1/1 -> Switch1/3
  Discharge Clock Reset/1 -> Subsystem1/1(Reset Order)
  Total Mass (Kg)/1 -> ?
  Product/1 -> Switch2/3  "Mass in Tank (Kg)"
  Product2/1 -> Product1/1
  Charge ON/1 -> Switch3/2
  Switch3/1 -> Product2/2
  Unit Delay1/1 -> Product2/1, Switch2/1
  Constant2/1 -> Switch3/3

== system Final_System_Model_V2/Tank Control ==
  note: This Block will be connected to the stateflow chart as to control the state of the tank, either it is:
      | a) Charging Only
      | b) Discharging Only
      | Or
      | c) Charging and Discharging at the same time
  Reset Charge Clock1 : Inport
  Reset Discharge Clock2 : Inport  Port=2
  Charging And Dicharging? : Constant  Value=0
  Charging oNLY : Constant  Value=0
  Constant1 : Constant  Value=0
  Pulse Generator : DiscretePulseGenerator  PulseType=Time based  Period=1  PulseWidth=5
  Switch : Switch  Criteria=u2 > Threshold
  trigger Pulse : Subsystem
  trigger Pulse1 : Subsystem
  Is Fuel Cell ON : Outport
  Reset Charge Clock : Outport  Port=2
  Out3 : Outport  Port=3
  Charging Only : Outport  Port=4
  wires:
  Pulse Generator/1 -> Switch/1
  Constant1/1 -> Is Fuel Cell ON/1
  Charging And Dicharging?/1 -> Switch/2
  Switch/1 -> Out3/1
  Charging oNLY/1 -> Charging Only/1
  Reset Charge Clock1/1 -> trigger Pulse/1(Trigger)
  trigger Pulse/1(Reset Charge Clock output) -> Reset Charge Clock/1
  trigger Pulse1/1(Reset Discharge Clock output) -> Switch/3
  Reset Discharge Clock2/1 -> trigger Pulse1/1(Trigger)

== system Final_System_Model_V2/180KW Fuel Cell Stack/From Load Current and Fuel Cell Output Current (A) to Valve Restriction Area (m^2) ==
  note: (3.0735e-14*(u(1)^3)) + (-5.0428e-11*(u(1)^2)) +(4.1772e-08*u(1)) + 2.7105e-07
  note: FEEDBACK BLOCK
  note: This block is the feedback block that controls the Flow control valve of the Hydrogen feeding system
      | I NPUTS: A) load Current (A) OUTPUTS: A) valve Restriction Area(m^2) as dictated by the Load Current
      | B) Output Current of the Fuel Cell (A) B) valve Restriction Area (m^2) as dictated by the Fuel Cell output current
  Load Profile Current (A) : Inport
  Output Current : Inport  Port=2
  Constant1 : Constant  Value=2.016e-3
  Constant2 : Constant  Value=96485
  Constant3 : Constant  Value=2
  Divide : Product  Inputs=*/
  Number Of Cells : Constant  Value=208
  Product : Product  Inputs=3
  Product1 : Product
  Subsystem : Subsystem
  Subsystem1 : Subsystem
  Valve Opening : Outport
  Valve Opening from Output Current : Outport  Port=2
  Hydrogen Mass Flow Rate (Kg/s) : Outport  Port=3
  wires:
  Output Current/1 -> Product/1, Subsystem/1(In1)
  Subsystem/1(Valve Opening from Output Current) -> Valve Opening from Output Current/1
  Load Profile Current (A)/1 -> Subsystem1/1(In1)
  Subsystem1/1(Out1) -> Valve Opening/1
  Product/1 -> Divide/1
  Number Of Cells/1 -> Product/2
  Constant1/1 -> Product/3
  Product1/1 -> Divide/2
  Constant3/1 -> Product1/2
  Constant2/1 -> Product1/1
  Divide/1 -> Hydrogen Mass Flow Rate (Kg/s)/1

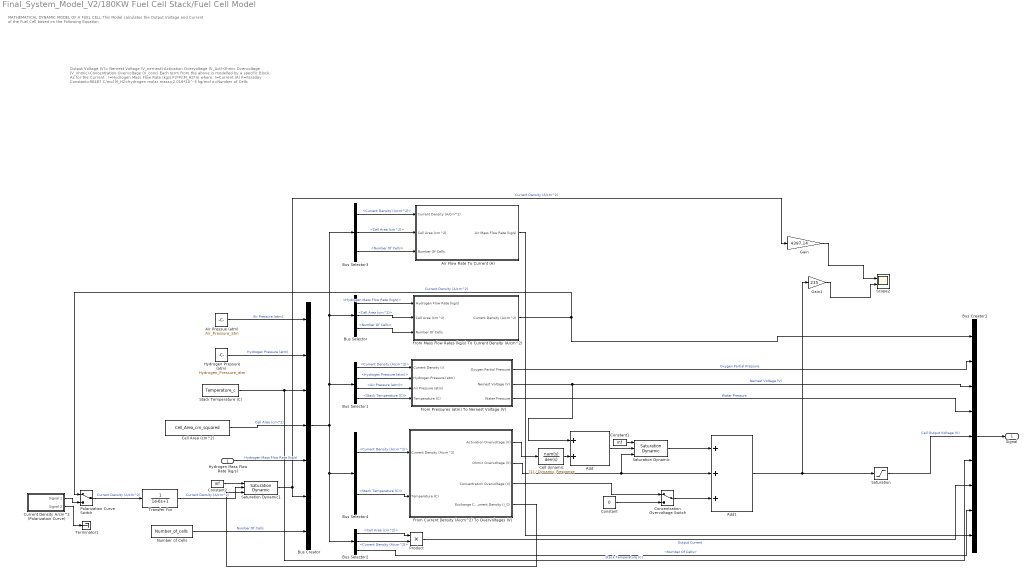
== system Final_System_Model_V2/180KW Fuel Cell Stack/Fuel Cell Model ==
  note: Output Voltage (V)= Nernest Voltage (V_nernest)-Activation Overvoltage (V_Act)-Ohmic Overvoltage (V_ohmic)-Concentration Overvoltage (V_conc)
      | Each term from the above is modelled by a specific Block.
      | As for the Current :
      |
      | I=Hydrogen Mass Flow Rate (kg/s)*2*F/(M_H2*n)
      | where: I=Current (A)
      | F=Faraday Constant=96487 C/mol
      | M_H2=hydrogen molar mass=2.016*10^-3 kg/mol
      | n=Number of Cells
  note: MATHEMATICAL DYNAMIC MODEL OF A FUEL CELL
      | This Model calculates the Output Voltage and Current of the Fuel Cell based on the Following Equation
  Hydrogen Mass Flow Rate (kg/s) : Inport
  " From Current Density (A/cm^2) To Overvoltages (V)" : Subsystem
  Add : Sum
  Add1 : Sum  Inputs=+++
  Air Flow Rate To Current (A) : Subsystem
  Air Pressue (atm) : Constant  Value=Air_Pressure_atm
  Bus Creator : BusCreator  Inputs=7
  Bus Creator1 : BusCreator  Inputs=9
  Bus Selector : BusSelector  OutputSignals=Hydrogen Mass Flow Rate (kg/s),Cell Area (cm^2),Number Of Cells
  Bus Selector1 : BusSelector  OutputSignals=Current Density (A/cm^2),Hydrogen Pressure (atm),Air Pressure (atm),Stack Temperature (C)
  Bus Selector2 : BusSelector  OutputSignals=Cell Area (cm^2),Current Density (A/cm^2),Number Of Cells
  Bus Selector3 : BusSelector  OutputSignals=Current Density (A/cm^2),Cell Area (cm^2),Number Of Cells
  Bus Selector4 : BusSelector  OutputSignals=Current Density (A/cm^2),Stack Temperature (C)
  Cell Area (cm^2) : Constant  Value=Cell_Area_cm_squared
  Cell dynamic : TransferFcn  Denominator=Dynamic_Response
  Concentration Overvoltage Switch : ManualSwitch
  Constant : Constant  Value=0
  Constant1 : Constant  Value=inf
  Constant2 : Constant  Value=inf
  Current Density A/cm^2 (Polarization Curve) : Subsystem  Tag=STV Subsys  LoadFcn=sigbuilder_block('load');  StartFcn=sigbuilder_block('start');  StopFcn=sigbuilder_block('stop');  ClipboardFcn=sigbuilder_block('clipboard');  mask(Sigbuilder block){tuvar=[0:10]}
      mask help: Simulink:masks:SigbuilderBlock_MD
      mask init:
      | if ~strcmp(get_param(bdroot(gcbh),'SimulationStatus'),'stopped') tuvar = sigbuilder_block('maskInit'); end
      settings: CopyFcn=sigbuilder_block('copy');  DeleteFcn=sigbuilder_block('delete');  ModelCloseFcn=sigbuilder_block('modelClose');  PreSaveFcn=sigbuilder_block('preSave');  PauseFcn=sigbuilder_block('pause');  ContinueFcn=sigbuilder_block('continue');  NameChangeFcn=sigbuilder_block('namechange');  OpenFcn=sigbuilder_block('open',[403.5 117 550.5 359.25 ]);  CloseFcn=sigbuilder_block('close');
      mask Display: plot(0, 0, 100, 100,[2, 2, 32, 32, 2], [68, 8, 8, 68, 68],[32, 2], [38, 38], [32, 19, 2],[53, 60, 44], [32, 17, 17, 2],[16, 16, 31, 31]);txt = getActiveGroup(gcbh);text(2, 100, txt,'verticalAlignment', 'top');
  From Mass Flow Rates (kg/s) To Current Density (A/cm^2) : Subsystem
  From Pressures (atm) To Nernest Voltage (V) : Subsystem
  Gain : Gain  Gain=4397.14
  Gain1 : Gain  Gain=235
  Hydrogen Pressure (atm) : Constant  Value=Hydrogen_Pressure_atm
  Number of Cells : Constant  Value=Number_of_cells
  Polarization Curve Switch : ManualSwitch
  Product : Product
  Saturation : Saturate  UpperLimit=inf  LowerLimit=0  ZeroCross=off
  Saturation Dynamic : simulink/Discontinuities/Saturation Dynamic  OutMin=[]  OutMax=[]  OutDataTypeStr=Inherit: Same as second input  OutDataType=sfix(16)  OutScaling=2^-10  DoSatur=off
  Saturation Dynamic1 : simulink/Discontinuities/Saturation Dynamic  OutMin=[]  OutMax=[]  OutDataTypeStr=Inherit: Same as second input  OutDataType=sfix(16)  OutScaling=2^-10  DoSatur=off
  Scope2 : Scope  NumInputPorts=2
  Stack Temperature (C) : Constant  Value=Temperature_c
  Terminator1 : Terminator
  Transfer Fcn : TransferFcn  Denominator=[1e-6 1]
  Signal : Outport
  wires:
  Saturation/1 -> Bus Creator1/5  "Cell Output Voltage (V)"
  Current Density A/cm^2 (Polarization Curve)/1(Signal 1) -> Polarization Curve Switch/2
  Hydrogen Mass Flow Rate (kg/s)/1 -> Bus Creator/5  "Hydrogen Mass Flow Rate (kg/s)"
  Bus Creator/1 -> Bus Selector2/1, Bus Selector4/1, Bus Selector1/1, Bus Selector3/1, Bus Selector/1
  From Mass Flow Rates (kg/s) To Current Density (A/cm^2)/1(Current Density (A/cm^2)) -> Bus Creator1/1, Polarization Curve Switch/1  "Current Density (A/cm^2)"
  Bus Selector/1 -> From Mass Flow Rates (kg/s) To Current Density (A/cm^2)/1(Hydrogen Flow Rate (kg/s))  "<Hydrogen Mass Flow Rate (kg/s)>"
  Bus Selector/2 -> From Mass Flow Rates (kg/s) To Current Density (A/cm^2)/2(Cell Area (cm^2))  "<Cell Area (cm^2)>"
  From Pressures (atm) To Nernest Voltage (V)/2(Nernest Voltage (V)) -> Bus Creator1/3, Add/1  "Nernest Voltage (V)"
  Bus Selector1/1 -> From Pressures (atm) To Nernest Voltage (V)/1(Current Density (i))  "<Current Density (A/cm^2)>"
  Bus Selector1/2 -> From Pressures (atm) To Nernest Voltage (V)/2(Hydrogen Pressure (atm))  "<Hydrogen Pressure (atm)>"
  Bus Selector1/3 -> From Pressures (atm) To Nernest Voltage (V)/3(Air Pressure (atm))  "<Air Pressure (atm)>"
  Bus Selector1/4 -> From Pressures (atm) To Nernest Voltage (V)/4(Temperature (C))  "<Stack Temperature (C)>"
  From Pressures (atm) To Nernest Voltage (V)/1(Oxygen Partial Pressure) -> Bus Creator1/2  "Oxygen Partial Pressure"
  From Pressures (atm) To Nernest Voltage (V)/3(Water Pressure) -> Bus Creator1/4  "Water Pressure"
  Bus Selector4/1 -> " From Current Density (A/cm^2) To Overvoltages (V)"/1(Current Density (A/cm^2))  "<Current Density (A/cm^2)>"
  Bus Selector4/2 -> " From Current Density (A/cm^2) To Overvoltages (V)"/2(Temperature (C))  "<Stack Temperature (C)>"
  " From Current Density (A/cm^2) To Overvoltages (V)"/1(Activation Overvoltage (V)) -> Cell dynamic/1
  Bus Creator1/1 -> Signal/1
  Polarization Curve Switch/1 -> Transfer Fcn/1  "Current Density (A/cm^2)"
  Constant2/1 -> Saturation Dynamic1/1
  " From Current Density (A/cm^2) To Overvoltages (V)"/4(Exchange Current Density (i_0)) -> Saturation Dynamic1/3
  Add1/1 -> Gain1/1, Saturation/1
  Cell dynamic/1 -> Add/2
  Add/1 -> Saturation Dynamic/2
  Constant1/1 -> Saturation Dynamic/1
  Saturation Dynamic/1 -> Add1/1
  " From Current Density (A/cm^2) To Overvoltages (V)"/3(Concentration Overvoltage (V)) -> Concentration Overvoltage Switch/1
  Bus Selector2/2 -> Product/2  "<Current Density (A/cm^2)>"
  Bus Selector2/1 -> Product/1  "<Cell Area (cm^2)>"
  Product/1 -> Bus Creator1/7  "Output Current"
  Bus Selector/3 -> From Mass Flow Rates (kg/s) To Current Density (A/cm^2)/3(Number Of Cells)  "<Number Of Cells>"
  Bus Selector2/3 -> Bus Creator1/8  "<Number Of Cells>"
  Saturation Dynamic1/1 -> Bus Creator/6, Gain/1  "Current Density (A/cm^2)"
  Transfer Fcn/1 -> Saturation Dynamic1/2  "Current Density (A/cm^2)"
  Stack Temperature (C)/1 -> Bus Creator/3, Bus Creator1/6  "Stack Temperature (C)"
  Hydrogen Pressure (atm)/1 -> Bus Creator/2  "Hydrogen Pressure (atm)"
  Air Pressue (atm)/1 -> Bus Creator/1  "Air Pressure (atm)"
  Number of Cells/1 -> Bus Creator/7  "Number Of Cells"
  Cell Area (cm^2)/1 -> Bus Creator/4  "Cell Area (cm^2)"
  " From Current Density (A/cm^2) To Overvoltages (V)"/2(Ohmic Overvoltage (V)) -> Saturation Dynamic/3, Add1/2
  Concentration Overvoltage Switch/1 -> Add1/3
  Constant/1 -> Concentration Overvoltage Switch/2
  Air Flow Rate To Current (A)/1(Air Mass Flow Rate (kg/s)) -> Bus Creator1/9
  Current Density A/cm^2 (Polarization Curve)/2(Signal 2) -> Terminator1/1
  Gain/1 -> Scope2/1
  Gain1/1 -> Scope2/2
  Bus Selector3/1 -> Air Flow Rate To Current (A)/1(Current Density (A/cm^2))  "<Current Density (A/cm^2)>"
  Bus Selector3/2 -> Air Flow Rate To Current (A)/2(Cell Area (cm^2))  "<Cell Area (cm^2)>"
  Bus Selector3/3 -> Air Flow Rate To Current (A)/3(Number Of Cells)  "<Number Of Cells>"
